simulink model "Regulator_continuu"  (R2023b)
settings: Solver=VariableStepAuto  StartTime=0.0  StopTime=300  RelTol=1e-3
values from neighbouring files (symbols this model uses):
  Kp = Vs/R    (= 0.45098)    [lab9.m]
  Tp = tt/3.9    (= 43.7820512821)    [lab9.m]
settings Model: Creator=Student13  LastModifiedBy=Student13

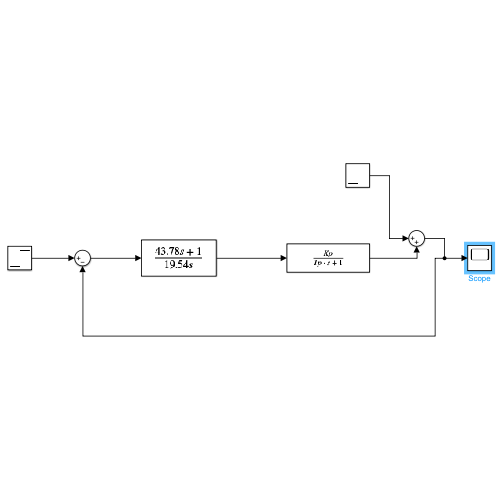
[thumbnail: Simulink's stored preview of the top-level diagram]
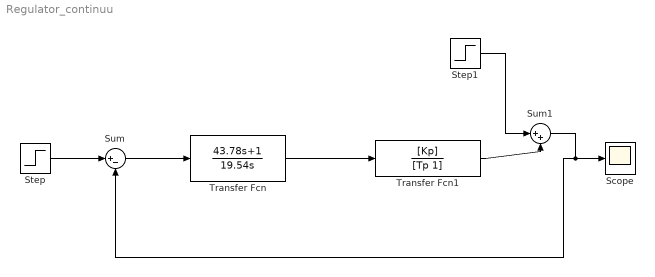
== system Regulator_continuu ==
  Scope : Scope
  Step : Step  Time=0  After=85  SampleTime=0
  Step1 : Step  Time=230  After=8  SampleTime=0
  Sum : Sum  Inputs=|+-
  Sum1 : Sum  Inputs=|++
  Transfer Fcn : TransferFcn  Numerator=[43.78 1]  Denominator=[19.54 0]
  Transfer Fcn1 : TransferFcn  Numerator=[Kp]  Denominator=[Tp 1]
  wires:
  Sum/1 -> Transfer Fcn/1
  Transfer Fcn/1 -> Transfer Fcn1/1
  Step/1 -> Sum/1
  Step1/1 -> Sum1/1
  Transfer Fcn1/1 -> Sum1/2
  Sum1/1 -> Scope/1, Sum/2
